simulink model "flight_simulator_glove"  (R2021a)
settings: Solver=VariableStepAuto  StartTime=0.0  StopTime=1000.0  RelTol=1e-3
libraries: aerolibfltsims x2, AE512Blockset x2, instrumentseriallib x2, mspfiltlib x1, sharedtransform x1
settings Model: Creator=maxab  LastModifiedBy=maxab

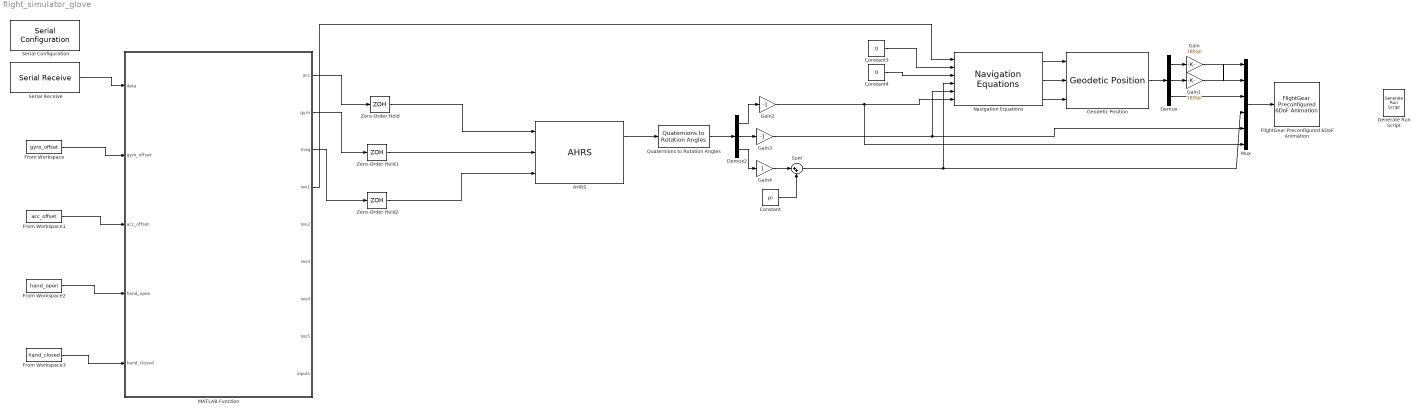
== system flight_simulator_glove ==
  AHRS : mspfiltlib/AHRS  DispRefFrame=NED  DecimationFactor=1  InitialProcessNoise=ahrsfilter.defaultProcessNoise  OrientationFormat=quaternion  SimulateUsing=Code generation  AccelerometerNoise=0.0001924722  GyroscopeNoise=9.1385e-5  MagnetometerNoise=0.1  GyroscopeDriftNoise=3.0462e-13  LinearAccelerationNoise=0.0096236100000000012  MagneticDisturbanceNoise=0.5  LinearAccelerationDecayFactor=0.5  MagneticDisturbanceDecayFactor=0.5  ExpectedMagneticFieldStrength=80
      settings: SourceProductBaseCode=TF,NV
  Constant : Constant  Value=pi
  Constant3 : Constant  Value=0
  Constant4 : Constant  Value=0
  Demux : Demux  Outputs=3
  Demux2 : Demux  Outputs=3
  FlightGear Preconfigured 6DoF Animation : aerolibfltsims/FlightGear Preconfigured 6DoF Animation  xFlightGearVersion=v2019.1  DestinationIpAddress=127.0.0.1  DestinationPort=5502  SampleTime=1/30  packetVersion=24
  From Workspace : FromWorkspace  VariableName=gyro_offset
  From Workspace1 : FromWorkspace  VariableName=acc_offset
  From Workspace2 : FromWorkspace  VariableName=hand_open
  From Workspace3 : FromWorkspace  VariableName=hand_closed
  Gain : Gain  Gain=180/pi
  Gain1 : Gain  Gain=180/pi
  Gain2 : Gain  Gain=-1
  Gain3 : Gain  Gain=-1
  Gain4 : Gain
  Generate Run Script : aerolibfltsims/Generate Run Script  Architecture=Win64  dataFlow=Send  GeometryModelName=c172p  AirportId=PHNL  RunwayId=08L  InitialAltitude=7224  InitialHeading=113  OffsetDistance=4.72  OffsetAzimuth=0  InstallScenery=off  DisableShaders=on  OriginAddress=127.0.0.1  DestinationPort=5502  OriginPort=5505  LocalAddress=127.0.0.1  OutputFileName=runfg.bat  FlightGearBaseDirectory=C:\Program Files\FlightGear 2020.3
  Geodetic Position : AE512Blockset/Geodetic Position  Xgeodetic0=Xgeodetic0
  MATLAB Function : MATLAB Function  TreatAsAtomicUnit=on
  Mux : Mux  Inputs=6
  Navigation Equations : AE512Blockset/Navigation Equations  Description=|
      | Version History  
      |                  
      | 05/24/05: Created
  Quaternions to Rotation Angles : sharedtransform/Quaternions to Rotation Angles  rotationOrder=ZYX  aMode=aMode
      settings: SourceProductBaseCode=AE,PW,DR,MT,UV,VE
  Serial Configuration : instrumentseriallib/Serial Configuration  Priority=-200000  Port=COM7  ComPort=COM7  BaudRate=38400  DataBits=8  Parity=none  StopBits=1  ByteOrder=little-endian  FlowControl=none  Timeout=10  SimulateUsing=Interpreted execution  BlockInModel=on
  Serial Receive : instrumentseriallib/Serial Receive  Priority=1  Port=COM7  ComPort=COM7  DataType=int16  SaveDataType=uint8  ToggleHeader=on  Header=[0xCA 0xFE]  ToggleTerminator=off  Terminator=<none>  CustomTerminator=[]  ToggleDataSize=on  DataSize=[13]  EnableBlockingMode=on  ActionDataUnavailable=Output last received value  ActionWhenDataUnavailable=Output last received value  CustomValue=0  SampleTime=0.05  SimulateUsing=Interpreted execution  BlockInModel=on
  Sum : Sum  Inputs=|++
  Zero-Order Hold : ZeroOrderHold  SampleTime=0.05
  Zero-Order Hold1 : ZeroOrderHold  SampleTime=0.05
  Zero-Order Hold2 : ZeroOrderHold  SampleTime=0.05
  wires:
  Mux/1 -> FlightGear Preconfigured 6DoF Animation/1
  Navigation Equations/1 -> Geodetic Position/1
  Navigation Equations/2 -> Geodetic Position/2
  Navigation Equations/3 -> Geodetic Position/3
  Geodetic Position/1 -> Demux/1
  Demux/1 -> Gain/1
  Demux/2 -> Gain1/1
  Gain1/1 -> Mux/1
  Gain/1 -> Mux/2
  Demux/3 -> Mux/3
  MATLAB Function/4(res1) -> Navigation Equations/1
  Constant3/1 -> Navigation Equations/2
  Constant4/1 -> Navigation Equations/3
  AHRS/1 -> Quaternions to Rotation Angles/1
  Zero-Order Hold2/1 -> AHRS/3
  Zero-Order Hold/1 -> AHRS/1
  Demux2/1 -> Gain2/1
  MATLAB Function/1(acc) -> Zero-Order Hold/1
  MATLAB Function/2(gyro) -> Zero-Order Hold1/1
  MATLAB Function/3(mag) -> Zero-Order Hold2/1
  Zero-Order Hold1/1 -> AHRS/2
  Quaternions to Rotation Angles/1 -> Demux2/1
  Demux2/2 -> Gain3/1
  From Workspace2/1 -> MATLAB Function/4(hand_open)
  From Workspace/1 -> MATLAB Function/2(gyro_offset)
  Serial Receive/1 -> MATLAB Function/1(data)
  From Workspace3/1 -> MATLAB Function/5(hand_closed)
  From Workspace1/1 -> MATLAB Function/3(acc_offset)
  Demux2/3 -> Gain4/1
  Gain2/1 -> Navigation Equations/6, Mux/6
  Gain3/1 -> Navigation Equations/5, Mux/5
  Sum/1 -> Navigation Equations/4, Mux/4
  Gain4/1 -> Sum/1
  Constant/1 -> Sum/2

== matlab function flight_simulator_glove/MATLAB Function ==
  data: acc output; gyro output; mag output; data input; gyro_offset input; acc_offset input; hand_open input; hand_closed input; res1 output; res2 output; res3 output; res4 output; res5 output; inputs output
function [acc, gyro, mag, res1, res2, res3, res4, res5, inputs] = fcn(data, gyro_offset, acc_offset, hand_open, hand_closed)
    usb_data = data';
    
    gyro_offset = double(gyro_offset');
    acc_offset = double(acc_offset');
    hand_open = double(hand_open');
    hand_closed = double(hand_closed');
        
    gyro = double(usb_data(4:6)) * (2000 * pi / (180 * 2^15)) - gyro_offset; % rad/s
    gyro(3) = gyro(3) * -1;
    acc = double(usb_data(1:3)) * 2 * 9.81 / (2^15) - acc_offset; % g-forces
    acc(3) = acc(3) * -1;
    mag = double(usb_data(10:12)) * 4 * 100 / (2^15); % microT
    
    res = [0 0 0 0 0];
    res(1) = bitand(int16(usb_data(8)), int16(hex2dec('00FF')), 'int16');
    res(2) = bitand(typecast(int16(usb_data(8)), "uint16"), uint16(hex2dec('FF00')), 'uint16');
    res(2) = bitshift(uint16(res(2)), -8, 'uint16'); % shift upper bits to lower place
    res(3) = bitand(int16(usb_data(9)), int16(hex2dec('00FF')), 'int16');
    res(4) = bitand(typecast(int16(usb_data(9)), "uint16"), uint16(hex2dec('FF00')), 'uint16');
    res(4) = bitshift(uint16(res(4)), -8, 'uint16'); % shift upper bits to lower place
    res(5) = bitand(int16(usb_data(10)), int16(hex2dec('00FF')), 'int16');
    
    norm_res = [0 0 0 0 0];
    for res_index=1:5
        norm_res(res_index) = (res(res_index) - hand_open(res_index)) * 200 / (hand_closed(res_index) - hand_open(res_index));
    end
    
    res1 = norm_res(1);
    res2 = norm_res(2);
    res3 = norm_res(3);
    res4 = norm_res(4);
    res5 = norm_res(5);
    
    inputs = bitand(int16(usb_data(10)), int16(hex2dec('FF00')), 'int16');
    inputs = bitshift(int16(inputs), -8, 'int16'); % shift upper bits to lower place

end
